simulink model "Ex2_B"  (R2021b)
settings: Solver=VariableStepAuto  StartTime=0.0  StopTime=10.0  RelTol=1e-3

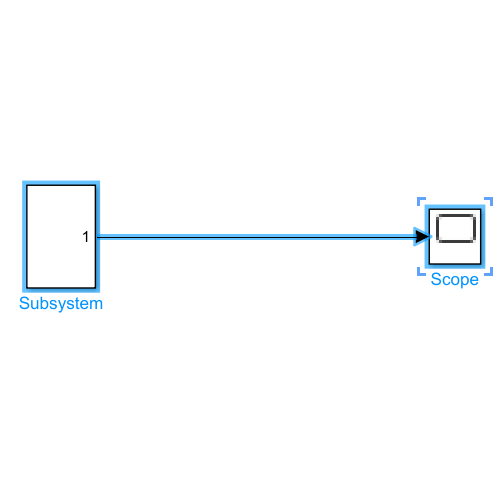
[thumbnail: Simulink's stored preview of the top-level diagram]
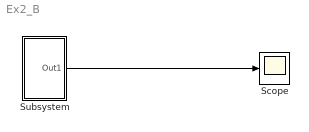
== system Ex2_B ==
  Scope : Scope
  Subsystem : Subsystem
  wires:
  Subsystem/1(Out1) -> Scope/1

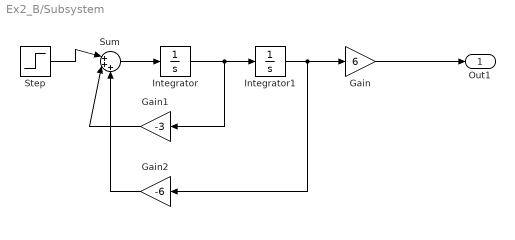
== system Ex2_B/Subsystem ==
  Gain : Gain  Gain=6
  Gain1 : Gain  Gain=-3
  Gain2 : Gain  Gain=-6
  Integrator : Integrator
  Integrator1 : Integrator
  Step : Step  SampleTime=0
  Sum : Sum  Inputs=|+++
  Out1 : Outport
  wires:
  Gain1/1 -> Sum/2
  Integrator/1 -> Gain1/1, Integrator1/1
  Sum/1 -> Integrator/1
  Gain2/1 -> Sum/3
  Integrator1/1 -> Gain2/1, Gain/1
  Step/1 -> Sum/1
  Gain/1 -> Out1/1
